simulink model "winter_simulink"  (R2022a)
settings: Solver=VariableStepAuto  StartTime=0  StopTime=stop_time  FixedStep=simulation.time_step_H  RelTol=1e-3
values from neighbouring files (symbols this model uses):
  Gc = 1/(1 + s*tau_c)    [PMSM_TF.m]    (also in PMSM_TF_pid.m; generator_test.m; tuning_example.m)
  GR = G*Riq_pid    [PMSM_TF.m]    (also in PMSM_TF_pid.m)
  I_eq = rotor.I + generator.I/gearbox.ratio^2    [parameters.m]
  lambda_vector = linspace(lambda_range(1), lambda_range(2), lambda_item)    [parameters.m]
  omega_rated = rated_values(2)    [parameters.m]
  pitch_range = deg2rad([-15 90])    [parameters.m]
  pitch_vector = linspace(pitch_range(1), pitch_range(2), pitch_item)    [parameters.m]
  rho = 1.225    [parameters.m]
  Riq = (Riq_pid.kp + Riq_pid.ki/s)    [PMSM_TF.m]    (also in PMSM_TF_pid.m = (Riq_pid.kp + Riq_pid.ki/s + Riq_pid.kd*s)*(1/(1 + s/(2*iq_o; generator_test.m = kiq_p + 1/s*kiq_i + s*kiq_d)
  Yiq = (B+s*I)/(L*I*s^2+(R*I+L*B)*s+R*B+1.5*(p*Lambda)^2)    [PMSM_TF.m]    (also in PMSM_TF_pid.m; generator_test.m; tuning_example.m)
undefined symbols (not defined in the file or in its folder): blade, gearbox, generator, lookup_cP, omega_R, rotor, simulation, wind
settings Model: Creator=Niccolò  LastModifiedBy=Niccolò

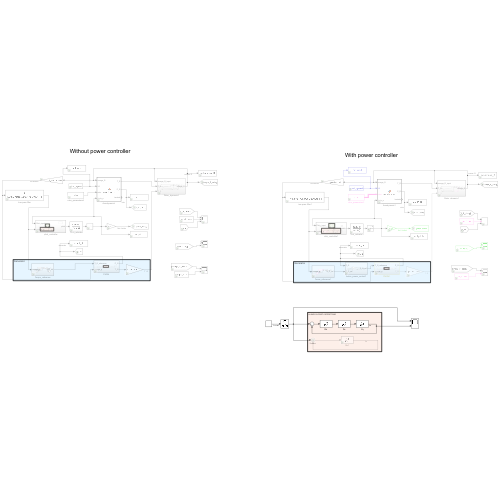
[thumbnail: Simulink's stored preview of the top-level diagram]
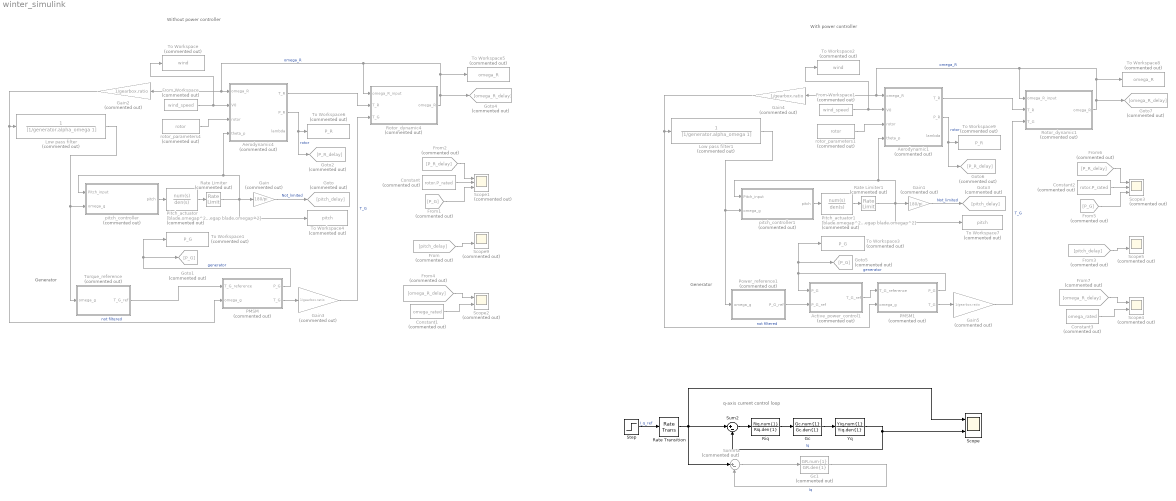
== system winter_simulink ==
  note: Without power controller
  note: Generator
  note: q-axis current control loop
  note: Generator
  note: With power controller
  Active_power_control1 : Subsystem  Commented=on
  Aerodynamic1 : MATLAB Function  Commented=on  TreatAsAtomicUnit=on
  Aerodynamic4 : MATLAB Function  Commented=on  TreatAsAtomicUnit=on
  Constant : Constant  Commented=on  Value=rotor.P_rated
  Constant1 : Constant  Commented=on  Value=omega_rated
  Constant2 : Constant  Commented=on  Value=rotor.P_rated
  Constant3 : Constant  Commented=on  Value=omega_rated
  From : From  Commented=on  GotoTag=pitch_delay
  From Workspace : FromWorkspace  Commented=on  VariableName=wind_speed  SampleTime=1/wind.sample_f
  From Workspace1 : FromWorkspace  Commented=on  VariableName=wind_speed  SampleTime=1/wind.sample_f
  From1 : From  Commented=on  GotoTag=P_G
  From2 : From  Commented=on  GotoTag=P_R_delay
  From3 : From  Commented=on  GotoTag=pitch_delay
  From4 : From  Commented=on  GotoTag=omega_R_delay
  From5 : From  Commented=on  GotoTag=P_G
  From6 : From  Commented=on  GotoTag=P_R_delay
  From7 : From  Commented=on  GotoTag=omega_R_delay
  Gain : Gain  Commented=on  Gain=180/pi  SampleTime=simulation.time_step_L
  Gain1 : Gain  Commented=on  Gain=180/pi  SampleTime=simulation.time_step_H
  Gain{2..5} (4 alike) : Gain  Commented=on  Gain=1/gearbox.ratio
  Gc : TransferFcn  Numerator=Gc.num{1}  Denominator=Gc.den{1}
  Gc1 : TransferFcn  Commented=on  Numerator=GR.num{1}  Denominator=GR.den{1}
  Goto : Goto  Commented=on  GotoTag=pitch_delay
  Goto1 : Goto  Commented=on  GotoTag=P_G
  Goto2 : Goto  Commented=on  GotoTag=P_R_delay
  Goto3 : Goto  Commented=on  GotoTag=pitch_delay
  Goto4 : Goto  Commented=on  GotoTag=omega_R_delay
  Goto5 : Goto  Commented=on  GotoTag=P_G
  Goto6 : Goto  Commented=on  GotoTag=P_R_delay
  Goto7 : Goto  Commented=on  GotoTag=omega_R_delay
  Low pass filter : TransferFcn  Commented=on  Denominator=[1/generator.alpha_omega 1]
  Low pass filter1 : TransferFcn  Commented=on  Denominator=[1/generator.alpha_omega 1]
  PMSM : Subsystem  Commented=on
  PMSM1 : Subsystem  Commented=on
  Pitch_actuator : TransferFcn  Commented=on  Numerator=[blade.omegap^2]  Denominator=[1 2*blade.zetap*blade.omegap blade.omegap^2]
  Pitch_actuator1 : TransferFcn  Commented=on  Numerator=[blade.omegap^2]  Denominator=[1 2*blade.zetap*blade.omegap blade.omegap^2]
  Power_reference1 : Subsystem  Commented=on
  Rate Limiter : RateLimiter  Commented=on  RisingSlewLimit=blade.pitch_rate  FallingSlewLimit=-blade.pitch_rate  SampleTimeMode=inherited
  Rate Limiter1 : RateLimiter  Commented=on  RisingSlewLimit=blade.pitch_rate  FallingSlewLimit=-blade.pitch_rate  SampleTimeMode=inherited
  Rate Transition : RateTransition  OutPortSampleTimeMultiple=1/10  OutPortSampleTime=simulation.time_step_L
  Riq : TransferFcn  Numerator=Riq.num{1}  Denominator=Riq.den{1}
  Rotor_dynamic1 : Subsystem  Commented=on
  Rotor_dynamic4 : Subsystem  Commented=on
  Scope : Scope  NumInputPorts=2
  Scope1 : Scope  Commented=on  NumInputPorts=3
  Scope{2,4..5,9} (4 alike) : Scope  Commented=on  NumInputPorts=2
  Scope3 : Scope  Commented=on  NumInputPorts=3
  Somma : Sum  Commented=on  Inputs=|+-
  Step : Step  SampleTime=simulation.time_step_H
  Sum2 : Sum  Inputs=|+-  SampleTime=simulation.time_step_L
  To Workspace : ToWorkspace  Commented=on  VariableName=wind  SaveFormat=Timeseries  SampleTime=-1
  To Workspace1 : ToWorkspace  Commented=on  VariableName=P_G  SaveFormat=Timeseries  SampleTime=-1
  To Workspace2 : ToWorkspace  Commented=on  VariableName=wind  SaveFormat=Timeseries  SampleTime=-1
  To Workspace3 : ToWorkspace  Commented=on  VariableName=P_G  SaveFormat=Timeseries  SampleTime=-1
  To Workspace4 : ToWorkspace  Commented=on  VariableName=pitch  SaveFormat=Timeseries  SampleTime=-1
  To Workspace5 : ToWorkspace  Commented=on  VariableName=omega_R  SaveFormat=Timeseries  SampleTime=-1
  To Workspace6 : ToWorkspace  Commented=on  VariableName=P_R  SaveFormat=Timeseries  SampleTime=-1
  To Workspace7 : ToWorkspace  Commented=on  VariableName=pitch  SaveFormat=Timeseries  SampleTime=-1
  To Workspace8 : ToWorkspace  Commented=on  VariableName=omega_R  SaveFormat=Timeseries  SampleTime=-1
  To Workspace9 : ToWorkspace  Commented=on  VariableName=P_R  SaveFormat=Timeseries  SampleTime=-1
  Torque_reference : Subsystem  Commented=on
  Yq : TransferFcn  Numerator=Yiq.num{1}  Denominator=Yiq.den{1}
  pitch_controller : Subsystem  Commented=on
  pitch_controller1 : Subsystem  Commented=on
  rotor_parameters1 : Constant  Commented=on  Value=rotor  OutDataTypeStr=Bus: rotor_bus
  rotor_parameters4 : Constant  Commented=on  Value=rotor  OutDataTypeStr=Bus: rotor_bus
  wires:
  Aerodynamic4/1(T_R) -> Rotor_dynamic4/2(T_R)
  From Workspace/1 -> To Workspace/1, Aerodynamic4/2(V0)
  rotor_parameters4/1 -> Aerodynamic4/3(rotor)
  Gain2/1 -> PMSM/2(omega_g), Low pass filter/1  "not filtered"
  Rotor_dynamic4/1(omega_R) -> Goto4/1, Gain2/1, Aerodynamic4/1(omega_R), Rotor_dynamic4/1(omega_R_input), To Workspace5/1  "omega_R"
  Aerodynamic4/2(P_R) -> Goto2/1, To Workspace6/1  "rotor"
  Gain/1 -> Goto/1  "Not_limited"
  PMSM/1(P_G) -> To Workspace1/1, Goto1/1  "generator"
  pitch_controller/1(pitch) -> Pitch_actuator/1
  PMSM/2(T_G) -> Gain3/1
  Gain3/1 -> Rotor_dynamic4/3(T_G)  "T_G"
  Step/1 -> Rate Transition/1  "I_q_ref"
  Gc/1 -> Yq/1
  Riq/1 -> Gc/1
  Yq/1 -> Scope/2, Sum2/2  "Iq"
  Sum2/1 -> Riq/1
  Low pass filter/1 -> Torque_reference/1(omega_g), pitch_controller/2(omega_g)
  Pitch_actuator/1 -> Rate Limiter/1
  Rate Limiter/1 -> Aerodynamic4/4(theta_p), pitch_controller/1(Pitch_input), Gain/1, To Workspace4/1
  From/1 -> Scope9/2
  From2/1 -> Scope1/1
  Constant/1 -> Scope1/2
  From4/1 -> Scope2/1
  From1/1 -> Scope1/3
  Constant1/1 -> Scope2/2
  Torque_reference/1(T_G_ref) -> PMSM/1(T_G_reference)
  From Workspace1/1 -> To Workspace2/1, Aerodynamic1/2(V0)
  Aerodynamic1/2(P_R) -> Goto6/1, To Workspace9/1  "rotor"
  From3/1 -> Scope5/2
  Gain4/1 -> PMSM1/2(omega_g), Low pass filter1/1  "not filtered"
  Rate Limiter1/1 -> Aerodynamic1/4(theta_p), pitch_controller1/1(Pitch_input), Gain1/1, To Workspace7/1
  pitch_controller1/1(pitch) -> Pitch_actuator1/1
  From6/1 -> Scope3/1
  Constant3/1 -> Scope4/2
  Constant2/1 -> Scope3/2
  From7/1 -> Scope4/1
  Low pass filter1/1 -> Power_reference1/1(omega_g), pitch_controller1/2(omega_g)
  Gain1/1 -> Goto3/1  "Not_limited"
  Gain5/1 -> Rotor_dynamic1/3(T_G)  "T_G"
  PMSM1/2(T_G) -> Gain5/1
  Aerodynamic1/1(T_R) -> Rotor_dynamic1/2(T_R)
  From5/1 -> Scope3/3
  rotor_parameters1/1 -> Aerodynamic1/3(rotor)
  PMSM1/1(P_G) -> Active_power_control1/1(P_G), To Workspace3/1, Goto5/1  "generator"
  Pitch_actuator1/1 -> Rate Limiter1/1
  Power_reference1/1(P_G_ref) -> Active_power_control1/2(P_G_ref)
  Active_power_control1/1(T_G_ref) -> PMSM1/1(T_G_reference)
  Rotor_dynamic1/1(omega_R) -> Goto7/1, Gain4/1, Aerodynamic1/1(omega_R), Rotor_dynamic1/1(omega_R_input), To Workspace8/1  "omega_R"
  Rate Transition/1 -> Somma/1, Sum2/1, Scope/1
  Somma/1 -> Gc1/1
  Gc1/1 -> Somma/2  "Iq"

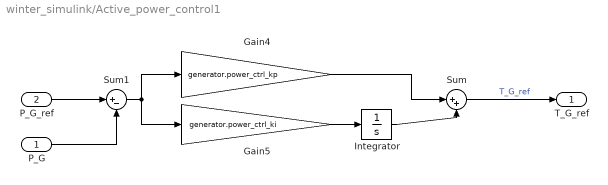
== system winter_simulink/Active_power_control1 ==
  P_G : Inport
  P_G_ref : Inport  Port=2
  Gain4 : Gain  Gain=generator.power_ctrl_kp
  Gain5 : Gain  Gain=generator.power_ctrl_ki
  Integrator : Integrator
  Sum : Sum  Inputs=|++
  Sum1 : Sum  Inputs=|+-
  T_G_ref : Outport
  wires:
  P_G/1 -> Sum1/2
  Gain5/1 -> Integrator/1
  Sum1/1 -> Gain4/1, Gain5/1
  Sum/1 -> T_G_ref/1  "T_G_ref"
  Gain4/1 -> Sum/1
  Integrator/1 -> Sum/2
  P_G_ref/1 -> Sum1/1

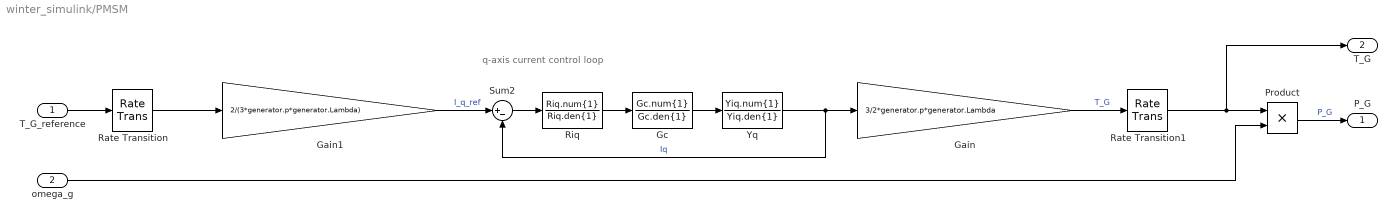
== system winter_simulink/PMSM ==
  note: q-axis current control loop
  T_G_reference : Inport
  omega_g : Inport  Port=2
  Gain : Gain  Gain=3/2*generator.p*generator.Lambda  SampleTime=simulation.time_step_L
  Gain1 : Gain  Gain=2/(3*generator.p*generator.Lambda)  SampleTime=simulation.time_step_L
  Gc : TransferFcn  Numerator=Gc.num{1}  Denominator=Gc.den{1}
  Product : Product
  Rate Transition : RateTransition  OutPortSampleTime=simulation.time_step_L
  Rate Transition1 : RateTransition
  Riq : TransferFcn  Numerator=Riq.num{1}  Denominator=Riq.den{1}
  Sum2 : Sum  Inputs=|+-  SampleTime=simulation.time_step_L
  Yq : TransferFcn  Numerator=Yiq.num{1}  Denominator=Yiq.den{1}
  P_G : Outport
  T_G : Outport  Port=2
  wires:
  Gc/1 -> Yq/1
  T_G_reference/1 -> Rate Transition/1
  Gain/1 -> Rate Transition1/1  "T_G"
  Riq/1 -> Gc/1
  Sum2/1 -> Riq/1
  Yq/1 -> Gain/1, Sum2/2  "Iq"
  Product/1 -> P_G/1  "P_G"
  omega_g/1 -> Product/2
  Gain1/1 -> Sum2/1  "I_q_ref"
  Rate Transition/1 -> Gain1/1
  Rate Transition1/1 -> T_G/1, Product/1

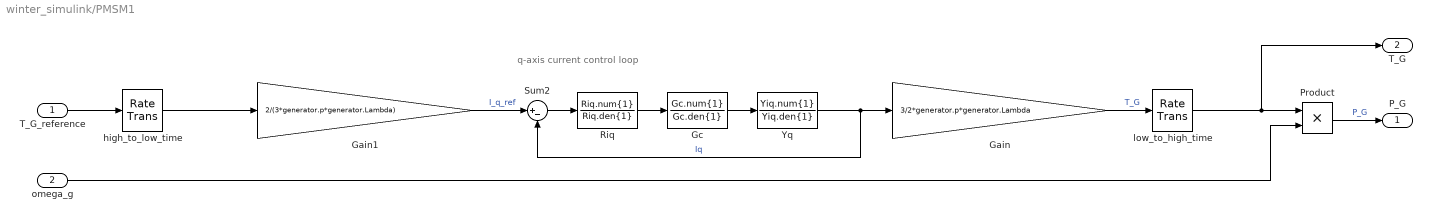
== system winter_simulink/PMSM1 ==
  note: q-axis current control loop
  T_G_reference : Inport
  omega_g : Inport  Port=2
  Gain : Gain  Gain=3/2*generator.p*generator.Lambda  SampleTime=simulation.time_step_L
  Gain1 : Gain  Gain=2/(3*generator.p*generator.Lambda)  SampleTime=simulation.time_step_L
  Gc : TransferFcn  Numerator=Gc.num{1}  Denominator=Gc.den{1}
  Product : Product
  Riq : TransferFcn  Numerator=Riq.num{1}  Denominator=Riq.den{1}
  Sum2 : Sum  Inputs=|+-  SampleTime=simulation.time_step_L
  Yq : TransferFcn  Numerator=Yiq.num{1}  Denominator=Yiq.den{1}
  high_to_low_time : RateTransition  OutPortSampleTime=simulation.time_step_L
  low_to_high_time : RateTransition
  P_G : Outport
  T_G : Outport  Port=2
  wires:
  Gc/1 -> Yq/1
  T_G_reference/1 -> high_to_low_time/1
  Gain/1 -> low_to_high_time/1  "T_G"
  Riq/1 -> Gc/1
  Sum2/1 -> Riq/1
  Yq/1 -> Gain/1, Sum2/2  "Iq"
  Product/1 -> P_G/1  "P_G"
  omega_g/1 -> Product/2
  Gain1/1 -> Sum2/1  "I_q_ref"
  high_to_low_time/1 -> Gain1/1
  low_to_high_time/1 -> T_G/1, Product/1

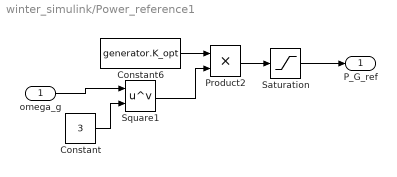
== system winter_simulink/Power_reference1 ==
  omega_g : Inport
  Constant : Constant  Value=3
  Constant6 : Constant  Value=generator.K_opt
  Product2 : Product
  Saturation : Saturate  UpperLimit=rotor.P_rated  LowerLimit=0
  Square1 : Math  Operator=pow
  P_G_ref : Outport
  wires:
  Product2/1 -> Saturation/1
  omega_g/1 -> Square1/1
  Square1/1 -> Product2/2
  Constant6/1 -> Product2/1
  Saturation/1 -> P_G_ref/1
  Constant/1 -> Square1/2

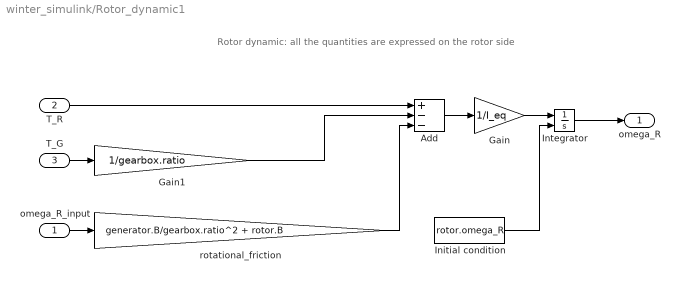
== system winter_simulink/Rotor_dynamic1 ==
  note: Rotor dynamic: all the quantities are expressed on the rotor side
  omega_R_input : Inport
  T_R : Inport  Port=2
  T_G : Inport  Port=3
  Add : Sum  Inputs=+--
  Gain : Gain  Gain=1/I_eq
  Gain1 : Gain  Gain=1/gearbox.ratio
  Initial condition : Constant  Value=rotor.omega_R
  Integrator : Integrator  InitialConditionSource=external  InitialCondition=omega_R
  rotational_friction : Gain  Gain=generator.B/gearbox.ratio^2 + rotor.B
  omega_R : Outport
  wires:
  Add/1 -> Gain/1
  Gain/1 -> Integrator/1
  T_R/1 -> Add/1
  Initial condition/1 -> Integrator/2
  omega_R_input/1 -> rotational_friction/1
  rotational_friction/1 -> Add/3
  T_G/1 -> Gain1/1
  Gain1/1 -> Add/2
  Integrator/1 -> omega_R/1

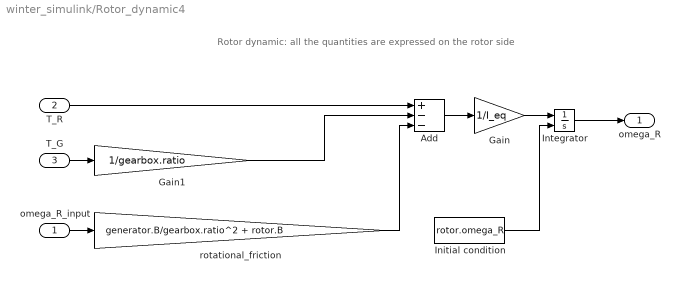
== system winter_simulink/Rotor_dynamic4 ==
  note: Rotor dynamic: all the quantities are expressed on the rotor side
  omega_R_input : Inport
  T_R : Inport  Port=2
  T_G : Inport  Port=3
  Add : Sum  Inputs=+--
  Gain : Gain  Gain=1/I_eq
  Gain1 : Gain  Gain=1/gearbox.ratio
  Initial condition : Constant  Value=rotor.omega_R
  Integrator : Integrator  InitialConditionSource=external  InitialCondition=omega_R
  rotational_friction : Gain  Gain=generator.B/gearbox.ratio^2 + rotor.B
  omega_R : Outport
  wires:
  Add/1 -> Gain/1
  Gain/1 -> Integrator/1
  T_R/1 -> Add/1
  Initial condition/1 -> Integrator/2
  omega_R_input/1 -> rotational_friction/1
  rotational_friction/1 -> Add/3
  T_G/1 -> Gain1/1
  Gain1/1 -> Add/2
  Integrator/1 -> omega_R/1

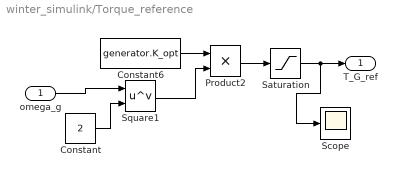
== system winter_simulink/Torque_reference ==
  omega_g : Inport
  Constant : Constant  Value=2
  Constant6 : Constant  Value=generator.K_opt
  Product2 : Product
  Saturation : Saturate  UpperLimit=rotor.P_rated*gearbox.ratio/omega_rated  LowerLimit=0
  Scope : Scope
  Square1 : Math  Operator=pow
  T_G_ref : Outport
  wires:
  Product2/1 -> Saturation/1
  omega_g/1 -> Square1/1
  Square1/1 -> Product2/2
  Constant6/1 -> Product2/1
  Saturation/1 -> Scope/1, T_G_ref/1
  Constant/1 -> Square1/2

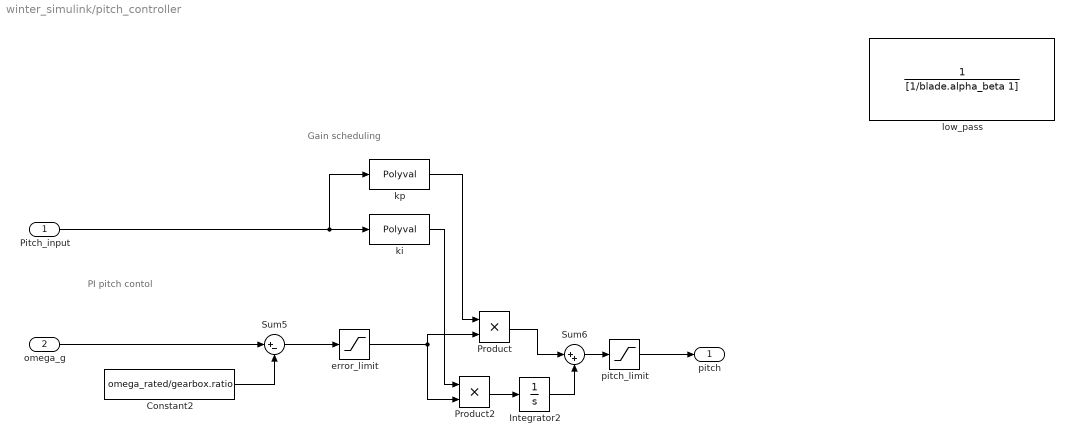
== system winter_simulink/pitch_controller ==
  note: Gain scheduling
  note: PI pitch contol
  Pitch_input : Inport
  omega_g : Inport  Port=2
  Constant2 : Constant  Value=omega_rated/gearbox.ratio
  Integrator2 : Integrator
  Product : Product
  Product2 : Product
  Sum5 : Sum  Inputs=|+-
  Sum6 : Sum  Inputs=|++
  error_limit : Saturate  UpperLimit=10  LowerLimit=-0.15
  ki : Polyval  Coefs=blade.ki_schedule
  kp : Polyval  Coefs=blade.kp_schedule
  low_pass : TransferFcn  Denominator=[1/blade.alpha_beta 1]
  pitch_limit : Saturate  UpperLimit=pitch_range(2)  LowerLimit=0
  pitch : Outport
  wires:
  Sum6/1 -> pitch_limit/1
  omega_g/1 -> Sum5/1
  Product/1 -> Sum6/1
  Constant2/1 -> Sum5/2
  ki/1 -> Product2/1
  kp/1 -> Product/1
  Pitch_input/1 -> kp/1, ki/1
  error_limit/1 -> Product2/2, Product/2
  Integrator2/1 -> Sum6/2
  Product2/1 -> Integrator2/1
  Sum5/1 -> error_limit/1
  pitch_limit/1 -> pitch/1

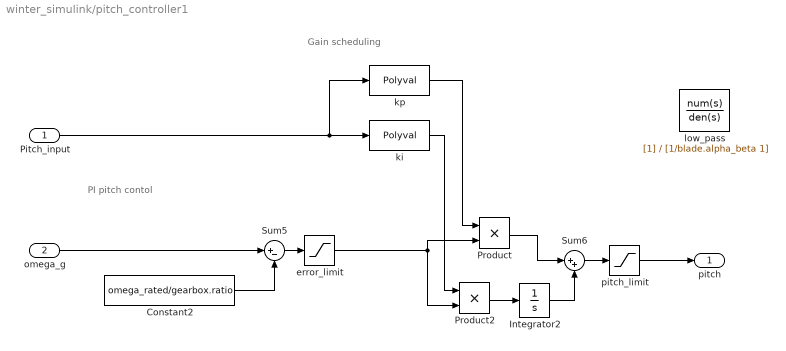
== system winter_simulink/pitch_controller1 ==
  note: Gain scheduling
  note: PI pitch contol
  Pitch_input : Inport
  omega_g : Inport  Port=2
  Constant2 : Constant  Value=omega_rated/gearbox.ratio
  Integrator2 : Integrator
  Product : Product
  Product2 : Product
  Sum5 : Sum  Inputs=|+-
  Sum6 : Sum  Inputs=|++
  error_limit : Saturate  UpperLimit=10  LowerLimit=-0.15
  ki : Polyval  Coefs=blade.ki_schedule
  kp : Polyval  Coefs=blade.kp_schedule
  low_pass : TransferFcn  Denominator=[1/blade.alpha_beta 1]
  pitch_limit : Saturate  UpperLimit=pitch_range(2)  LowerLimit=0
  pitch : Outport
  wires:
  Sum6/1 -> pitch_limit/1
  omega_g/1 -> Sum5/1
  Product/1 -> Sum6/1
  Constant2/1 -> Sum5/2
  ki/1 -> Product2/1
  kp/1 -> Product/1
  Pitch_input/1 -> kp/1, ki/1
  error_limit/1 -> Product2/2, Product/2
  Integrator2/1 -> Sum6/2
  Product2/1 -> Integrator2/1
  Sum5/1 -> error_limit/1
  pitch_limit/1 -> pitch/1

== matlab function winter_simulink/Aerodynamic4 ==
  data: omega_R input; V0 input; T_R output; P_R output; rho parameter; rotor input; theta_p input; lambda_vector parameter; pitch_vector parameter; lookup_cP parameter; lambda output
function [T_R, P_R, lambda] = Aerodynamic(omega_R, V0, rho, rotor, ...
  theta_p, lambda_vector, pitch_vector, lookup_cP) 

R = rotor.R;                  % rotor radius [m]

% retrive the cP from the look-up table
lambda = omega_R*R/V0;                                                
cP = interp2(lambda_vector, pitch_vector, lookup_cP, lambda, theta_p);

P_R = 0.5*rho*V0^3*pi*R^2*cP; % rotor power [W]
T_R = P_R/omega_R;            % rotor torque [Nm]

== matlab function winter_simulink/Aerodynamic1 ==
  data: omega_R input; V0 input; T_R output; P_R output; rho parameter; rotor input; theta_p input; lambda_vector parameter; pitch_vector parameter; lookup_cP parameter; lambda output
function [T_R, P_R, lambda] = Aerodynamic(omega_R, V0, rho, rotor, ...
  theta_p, lambda_vector, pitch_vector, lookup_cP) 

R = rotor.R;                  % rotor radius [m]

% retrive the cP from the look-up table
lambda = omega_R*R/V0;                                                
cP = interp2(lambda_vector, pitch_vector, lookup_cP, lambda, theta_p);

P_R = 0.5*rho*V0^3*pi*R^2*cP; % rotor power [W]
T_R = P_R/omega_R;            % rotor torque [Nm]
